simulink model "LQR_ctrl"  (R2025b)
settings: Solver=VariableStepAuto  StartTime=0.0  StopTime=20  RelTol=1e-3
values from neighbouring files (symbols this model uses):
  A = [0 1 0 0;     (m_b*g*r^2)/(I_b*l) 0 (m_b*g*r^2)/(I_b) 0 ;      0 0 0 1;    20 0 (M_r*d*g)/I_r 0 ]    [Copy_of_LQR_ctrl.m]    (also in LQR_ctrl.m = [0 1 0 0;     A1(1,1) 0 A1(1,2) 0;     0 0 0 1;     A1(2,1) ; Rlocus_ctrl.m = [0 1 0 0;     A1(1,1) 0 A1(1,2) 0;     0 0 0 1;     A1(2,1) ; State4.m = [0 1 0 0;     A1(1,1) 0 A1(1,2) 0;     0 0 0 1;     A1(2,1) ; pole_placement_ctrl.m = [0 1 0 0;     A1(1,1) 0 0 0;     0 0 0 1;    A1(2,1) 0 A1(2,)
  B = -[0 ; 0; 0 ; ((I_w/R) + (M_w+M_r)*R)/(I_r)]    [Copy_of_LQR_ctrl.m]    (also in LQR_ctrl.m = -[0 ; B1(1); 0 ; B1(2)]; Rlocus_ctrl.m = -[0 ; B1(1); 0 ; B1(2)]; State4.m = -[0 ; B1(1); 0 ; B1(2)]; pole_placement_ctrl.m = -[0 ; B1(1); 0 ; B1(2)])
  K = lqr(A, B, Q, R)    [State4.m]    (also in pole_placement_ctrl.m = place(A,B,poles))
  x0 = [0.01, 0, deg2rad(5),0]'    [Copy_of_LQR_ctrl.m]    (also in LQR_ctrl.m; State4.m = x0 - x_ref; pole_placement_ctrl.m = [0.005, 0, deg2rad(0.2),0]')
settings Model: Creator=Abhi  LastModifiedBy=Abhi

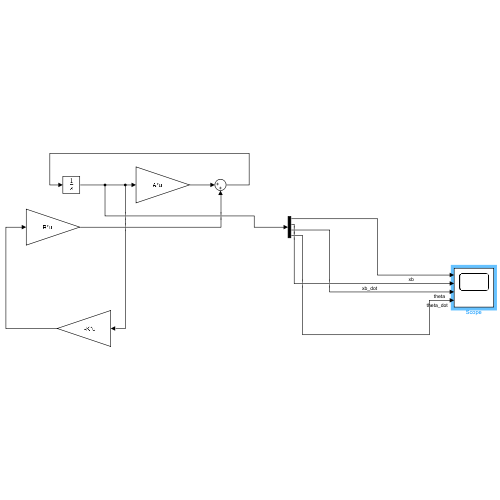
[thumbnail: Simulink's stored preview of the top-level diagram]
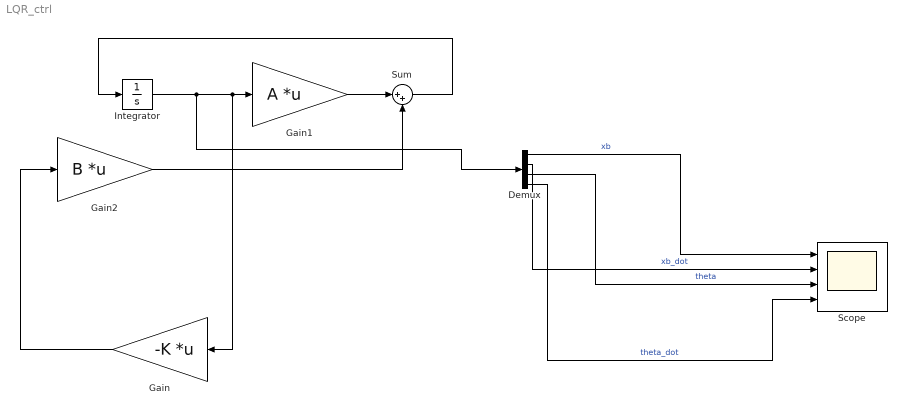
== system LQR_ctrl ==
  Demux : Demux
  Gain : Gain  Gain=-K  Multiplication=Matrix(K*u)
  Gain1 : Gain  Gain=A  Multiplication=Matrix(K*u)
  Gain2 : Gain  Gain=B  Multiplication=Matrix(K*u)
  Integrator : Integrator  InitialCondition=x0
  Scope : Scope  NumInputPorts=4
      settings: SampleTime=1e-4  ActiveDisplayYMinimum=-0.0076623295155117139  ActiveDisplayYMaximum=0.01196248105727908
  Sum : Sum  Inputs=|++
  wires:
  Gain/1 -> Gain2/1
  Gain1/1 -> Sum/1
  Demux/3 -> Scope/3  "theta"
  Demux/1 -> Scope/1  "xb"
  Demux/4 -> Scope/4  "theta_dot"
  Demux/2 -> Scope/2  "xb_dot"
  Integrator/1 -> Demux/1, Gain/1, Gain1/1
  Gain2/1 -> Sum/2
  Sum/1 -> Integrator/1
